simulink subsystem "kls_can_interface"  (R2024b)
settings: Solver=VariableStepAuto  StartTime=0.0  StopTime=10.0  RelTol=1e-3
libraries: c280xlib x2, svdutilitieslib x2
settings Model: Creator=orang  LastModifiedBy=orang

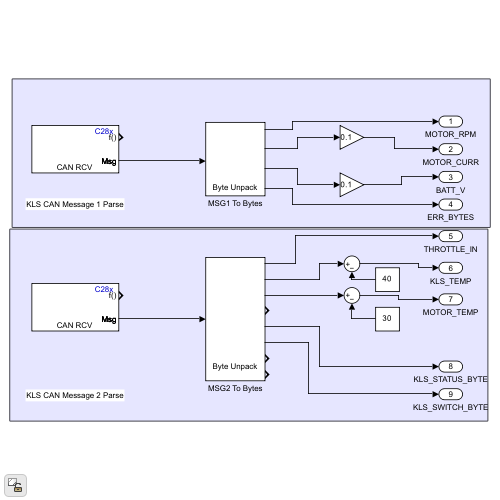
[thumbnail: Simulink's stored preview of the top-level diagram]
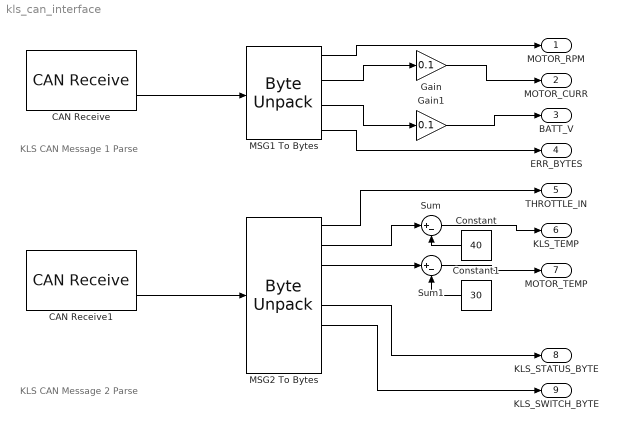
== system kls_can_interface ==
  note: KLS CAN Message 2 Parse
  note: KLS CAN Message 1 Parse
  CAN Receive : c280xlib/CAN Receive  chipFamily=C280x  useModule=CAN_A  mailboxNo=0  messageID=hex2dec('0CF11E05')  messageType=Extended (29-bit identifier)  enableAcceptanceFiltering=off  messageIDMask=0  sampleTime=0.05  dataType=uint8  outputAction=Output last received values  initValue=0  outputMessageID=off  outputMessageLength=off  outputMessageTimeStamp=off  postInterrupt=off  interruptLine=0
      settings: LibrarySourceBlock=c2837xDlib/CAN Receive
  CAN Receive1 : c280xlib/CAN Receive  chipFamily=C280x  useModule=CAN_A  mailboxNo=1  messageID=hex2dec('0CF11F05')  messageType=Extended (29-bit identifier)  enableAcceptanceFiltering=off  messageIDMask=0  sampleTime=0.05  dataType=uint8  outputAction=Output last received values  initValue=0  outputMessageID=off  outputMessageLength=off  outputMessageTimeStamp=off  postInterrupt=off  interruptLine=0
      settings: LibrarySourceBlock=c2837xDlib/CAN Receive
  Constant : Constant  Value=40
  Constant1 : Constant  Value=30
  Gain : Gain  Gain=0.1
  Gain1 : Gain  Gain=0.1
  MSG1 To Bytes : svdutilitieslib/Byte Unpack  dimensions={[1],[1],[1],[1]}  datatypes={'uint16','uint16','uint16','uint16'}  byteAlign=1  blockPlatform=tic2000
      settings: LibrarySourceBlock=c2000lib/Target Communication/Byte Unpack
  MSG2 To Bytes : svdutilitieslib/Byte Unpack  dimensions={[1],[1],[1],[1],[1],[1],[1],[1]}  datatypes={'uint8','uint8','uint8','uint8','uint8','uint8','uint8','uint8'}  byteAlign=1  blockPlatform=tic2000
      settings: LibrarySourceBlock=c2000lib/Target Communication/Byte Unpack
  Sum : Sum  Inputs=|+-
  Sum1 : Sum  Inputs=|+-
  MOTOR_RPM : Outport
  MOTOR_CURR : Outport  Port=2
  BATT_V : Outport  Port=3
  ERR_BYTES : Outport  Port=4
  THROTTLE_IN : Outport  Port=5
  KLS_TEMP : Outport  Port=6
  MOTOR_TEMP : Outport  Port=7
  KLS_STATUS_BYTE : Outport  Port=8
  KLS_SWITCH_BYTE : Outport  Port=9
  wires:
  CAN Receive/2 -> MSG1 To Bytes/1
  CAN Receive1/2 -> MSG2 To Bytes/1
  MSG1 To Bytes/1 -> MOTOR_RPM/1
  MSG1 To Bytes/2 -> Gain/1
  MSG1 To Bytes/3 -> Gain1/1
  MSG1 To Bytes/4 -> ERR_BYTES/1
  MSG2 To Bytes/1 -> THROTTLE_IN/1
  MSG2 To Bytes/2 -> Sum/1
  Constant/1 -> Sum/2
  Sum/1 -> KLS_TEMP/1
  MSG2 To Bytes/3 -> Sum1/1
  Constant1/1 -> Sum1/2
  Sum1/1 -> MOTOR_TEMP/1
  MSG2 To Bytes/5 -> KLS_STATUS_BYTE/1
  MSG2 To Bytes/6 -> KLS_SWITCH_BYTE/1
  Gain/1 -> MOTOR_CURR/1
  Gain1/1 -> BATT_V/1
